simulink model "ver1_real_discrete"  (R2018b)
settings: Solver=FixedStepAuto  StartTime=0.0  StopTime=100  FixedStep=10e-3  RelTol=1e-3
InitFcn:
  | ver1_real_pendulum
values from neighbouring files (symbols this model uses):
  A_new = [A, zeros(2,1) ... (first row only)    [PendulumSS.m]    (also in ver1_real_pendulum.m = [A,zeros(2,1))
  B_new = [B ... (first row only)    [PendulumSS.m]    (also in ver1_real_pendulum.m)
  E = [0 ... (first row only)    [ver1_real_pendulum.m]
  Init_condition = [0 ... (first row only)    [ver1_real_pendulum.m]
  K = place(A_new,B_new,p)    [PendulumSS.m]    (also in ver1_real_pendulum.m = dlqr(A_new,B_new,Q,R))
  Ts = 0.03    [ver1_real_pendulum.m]
settings Model: Creator=Mehmet  LastModifiedBy=Seko
settings SFSimCC: SimUseLocalCustomCode=off
settings RTWCC: RTWUseLocalCustomCode=off

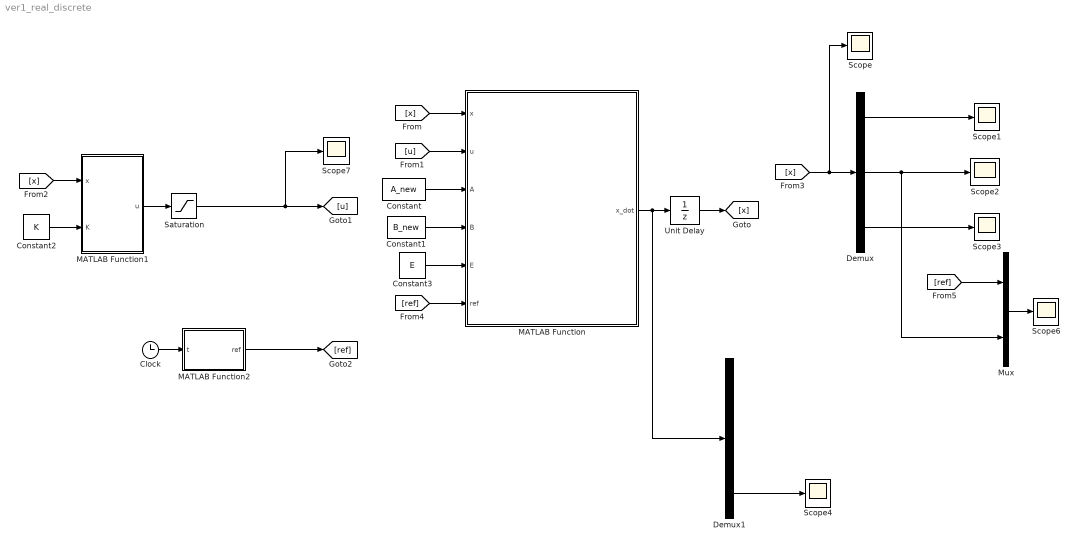
== system ver1_real_discrete ==
  Clock : Clock
  Constant : Constant  Value=A_new  VectorParams1D=off
  Constant1 : Constant  Value=B_new  VectorParams1D=off
  Constant2 : Constant  Value=K  VectorParams1D=off
  Constant3 : Constant  Value=E  VectorParams1D=off
  Demux : Demux  Outputs=3
  Demux1 : Demux  Outputs=3
  MATLAB Function : MATLAB Function  TreatAsAtomicUnit=on
  MATLAB Function1 : MATLAB Function  TreatAsAtomicUnit=on
  MATLAB Function2 : MATLAB Function  TreatAsAtomicUnit=on
  Mux : Mux  Inputs=2
  Saturation : Saturate  UpperLimit=6  LowerLimit=-6
  Scope{,1..4,6..7} (7 alike) : Scope
  Unit Delay : UnitDelay  InitialCondition=Init_condition  SampleTime=Ts
  wires:
  MATLAB Function/1(x_dot) -> Demux1/1, Unit Delay/1
  Unit Delay/1 -> [x]
  [x] -> MATLAB Function/1(x)
  [u] -> MATLAB Function/2(u)
  Constant/1 -> MATLAB Function/3(A)
  Constant1/1 -> MATLAB Function/4(B)
  [x] -> MATLAB Function1/1(x)
  Constant2/1 -> MATLAB Function1/2(K)
  [x] -> Scope/1, Demux/1
  Demux/1 -> Scope1/1
  Demux/2 -> Mux/2, Scope2/1
  Demux/3 -> Scope3/1
  Constant3/1 -> MATLAB Function/5(E)
  Clock/1 -> MATLAB Function2/1(t)
  [ref] -> MATLAB Function/6(ref)
  [ref] -> Mux/1
  Mux/1 -> Scope6/1
  MATLAB Function1/1(u) -> Saturation/1
  MATLAB Function2/1(ref) -> [ref]
  Demux1/3 -> Scope4/1
  Saturation/1 -> Scope7/1, [u]

== matlab function ver1_real_discrete/MATLAB Function1 ==
  data: x input; u output; K input
function u = fcn(x,K)

u_int = -K*x;

% if abs(u_int) < (20*3.36*10^-3) && u_int > 0
% 
%     u_int = (20*3.36*10^-3);
%     
% end
% 
% if abs(u_int) < (20*3.36*10^-3) && u_int < 0
% 
%     u_int = -(20*3.36*10^-3);
%     
% end


% if abs(u_int) < (20*10^-3)
% 
%     u_int = 0;
%     
% end

u = u_int;

== matlab function ver1_real_discrete/MATLAB Function ==
  data: x input; u input; x_dot output; A input; B input; E input; ref input
function x_dot = fcn(x,u,A,B,E,ref)

% output
x_dot = A*x + B*u + E*ref;

end

== matlab function ver1_real_discrete/MATLAB Function2 ==
  data: t input; ref output
function ref = fcn(t)


f = 0.2;

A = 300*0.088*pi/180;
B = 0;

ref = A*sin(2*pi*f*t) + B;
%ref=2;
end
